simulink model "PlantModels2"  (R2024a)
settings: Solver=VariableStepAuto  StartTime=0.0  StopTime=10.0  RelTol=1e-3
model workspace (MAT data in the model file):
  A = [0  1  0; 0  0  1; 0  -2.65135135135  0]
  B = [0; 0; 1]
  C = [2.65135135135 0 0]
  g = 9.81
  l = 3.7
settings Model: Creator=Riley  LastModifiedBy=Riley

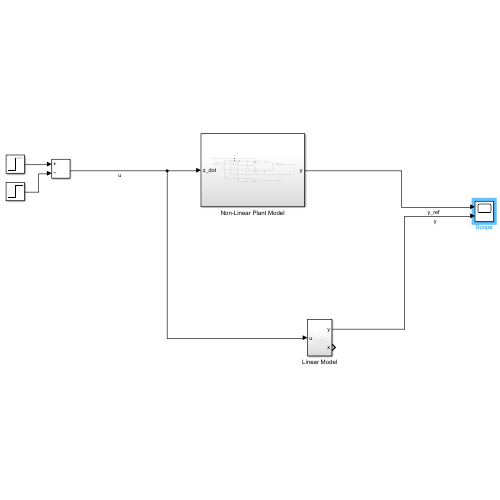
[thumbnail: Simulink's stored preview of the top-level diagram]
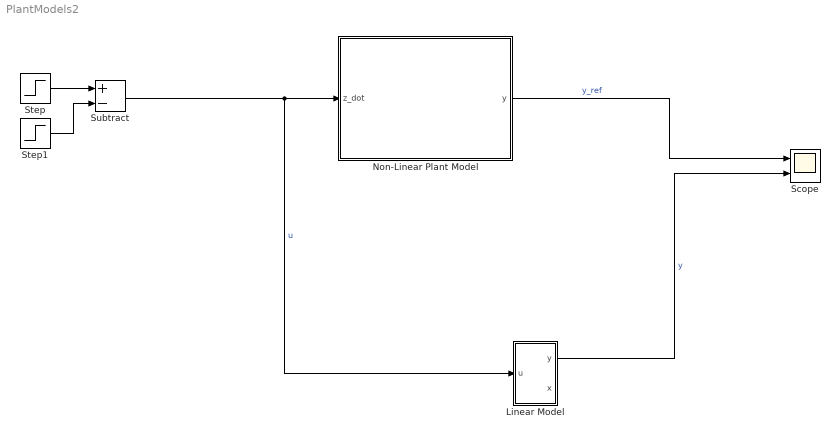
== system PlantModels2 ==
  Linear Model : Subsystem
  Non-Linear Plant Model : Subsystem
  Scope : Scope  NumInputPorts=2
  Step : Step  Time=0  SampleTime=0
  Step1 : Step  SampleTime=0
  Subtract : Sum  Inputs=+-
  wires:
  Step/1 -> Subtract/1
  Step1/1 -> Subtract/2
  Subtract/1 -> Linear Model/1(u), Non-Linear Plant Model/1(z_dot)  "u"
  Non-Linear Plant Model/1(y) -> Scope/1  "y_ref"
  Linear Model/1(y) -> Scope/2  "y"

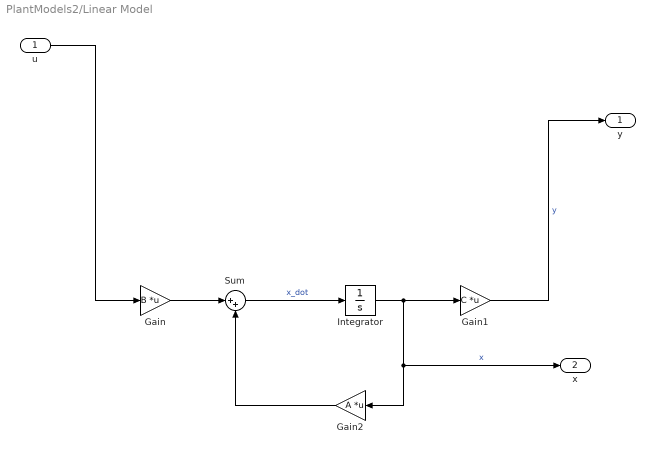
== system PlantModels2/Linear Model ==
  u : Inport
  Gain : Gain  Gain=B  Multiplication=Matrix(K*u)
  Gain1 : Gain  Gain=C  Multiplication=Matrix(K*u)
  Gain2 : Gain  Gain=A  Multiplication=Matrix(K*u)
  Integrator : Integrator
  Sum : Sum  Inputs=|++
  y : Outport
  x : Outport  Port=2
  wires:
  Sum/1 -> Integrator/1  "x_dot"
  Integrator/1 -> x/1, Gain2/1, Gain1/1  "x"
  Gain/1 -> Sum/1
  u/1 -> Gain/1
  Gain2/1 -> Sum/2
  Gain1/1 -> y/1  "y"

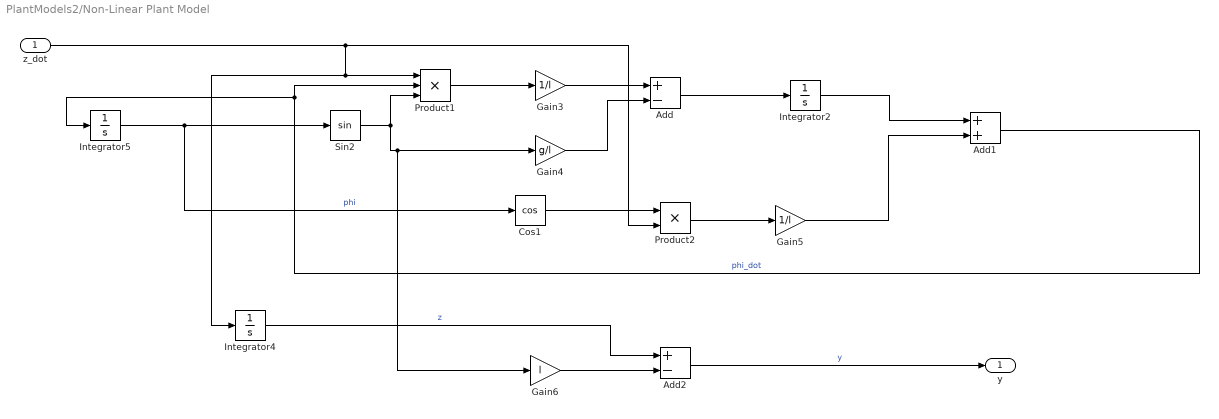
== system PlantModels2/Non-Linear Plant Model ==
  z_dot : Inport
  Add : Sum  Inputs=+-
  Add1 : Sum
  Add2 : Sum  Inputs=+-
  Cos1 : Trigonometry  Operator=cos
  Gain3 : Gain  Gain=1/l
  Gain4 : Gain  Gain=g/l
  Gain5 : Gain  Gain=1/l
  Gain6 : Gain  Gain=l
  Integrator2 : Integrator
  Integrator4 : Integrator
  Integrator5 : Integrator
  Product1 : Product  Inputs=3
  Product2 : Product
  Sin2 : Trigonometry
  y : Outport
  wires:
  z_dot/1 -> Integrator4/1, Product1/1, Product2/2
  Sin2/1 -> Gain4/1, Gain6/1, Product1/3
  Product1/1 -> Gain3/1
  Add1/1 -> Product1/2, Integrator5/1  "phi_dot"
  Gain3/1 -> Add/1
  Integrator5/1 -> Cos1/1, Sin2/1  "phi"
  Integrator2/1 -> Add1/1
  Add/1 -> Integrator2/1
  Cos1/1 -> Product2/1
  Product2/1 -> Gain5/1
  Gain4/1 -> Add/2
  Gain5/1 -> Add1/2
  Gain6/1 -> Add2/2
  Integrator4/1 -> Add2/1  "z"
  Add2/1 -> y/1  "y"
